simulink model "kalman_filter_state_est"  (R2024a)
settings: Solver=VariableStepAuto  StartTime=0.0  StopTime=10.0  RelTol=1e-3
undefined symbols (not defined in the file): b, Continuous, J, K, Kc, L, R, Time
libraries: simulink x3, ctrlSharedLib x1
settings Model: Creator=Harish  LastModifiedBy=Harish

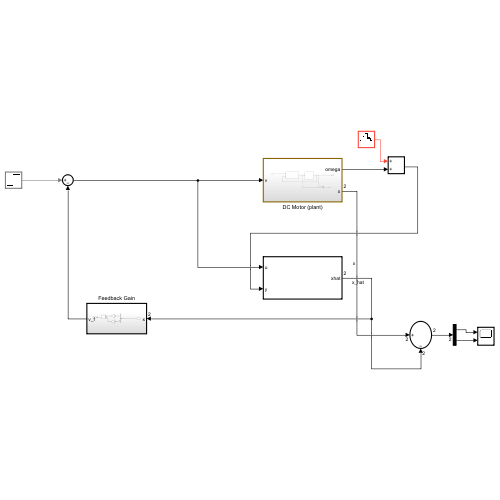
[thumbnail: Simulink's stored preview of the top-level diagram]
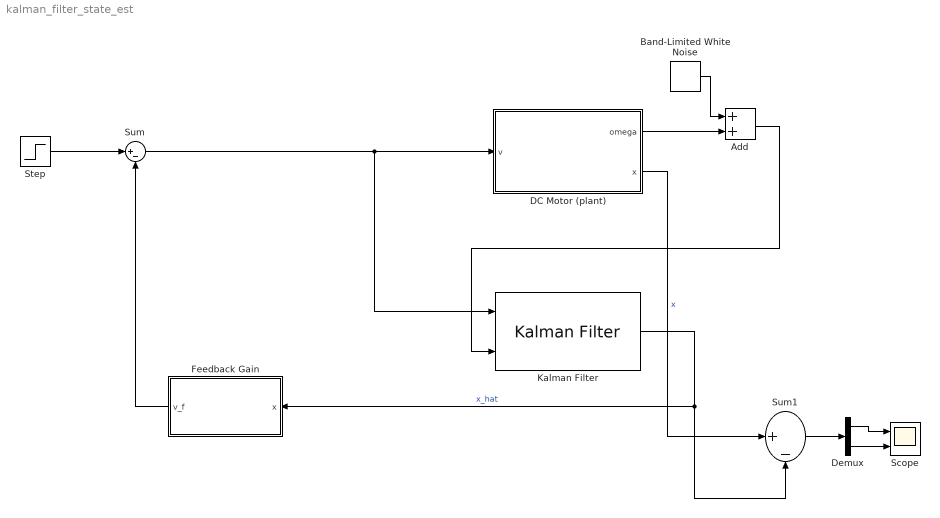
== system kalman_filter_state_est ==
  Add : Sum
  Band-Limited White Noise : simulink/Sources/Band-Limited White Noise  Cov=0.01  Ts=0.01  seed=0
  DC Motor (plant) : Subsystem
  Demux : Demux  Outputs=2
  Feedback Gain : Subsystem
  Kalman Filter : ctrlSharedLib/Kalman Filter  TimeDomain=Continuous-Time  UseCurrentEstimator=on  ModelSource=LTI State-Space Variable  ModelSourceVariable=dcMotorSS  A=0.95  B=1  C=1  D=0  NumberOfStates=1  NumberOfInputs=1  NumberOfOutputs=1  InitialEstimateSource=Dialog  X0=0  P0=10  UseK=off  UseGH=off  NumberOfProcessNoiseInputs=1  G=1  TimeInvariantG=on  H=0  TimeInvariantH=on  Q=10  TimeInvariantQ=on  R=1  TimeInvariantR=on  N=0  TimeInvariantN=on  AddInputPort=on  AddEnablePort=off  OutputEstimatedY=off  OutputP=off  Ts=-1
  Scope : Scope  NumInputPorts=2
  Step : Step  SampleTime=0
  Sum : Sum  Inputs=|+-
  Sum1 : Sum  Inputs=|+-
  wires:
  DC Motor (plant)/1(omega) -> Add/2
  Step/1 -> Sum/1
  Feedback Gain/1(v_f) -> Sum/2
  Kalman Filter/1 -> Sum1/2, Feedback Gain/1(x)  "x_hat"
  Band-Limited White Noise/1 -> Add/1
  Add/1 -> Kalman Filter/2
  DC Motor (plant)/2(x) -> Sum1/1  "x"
  Sum/1 -> Kalman Filter/1, DC Motor (plant)/1(v)
  Sum1/1 -> Demux/1
  Demux/1 -> Scope/1
  Demux/2 -> Scope/2

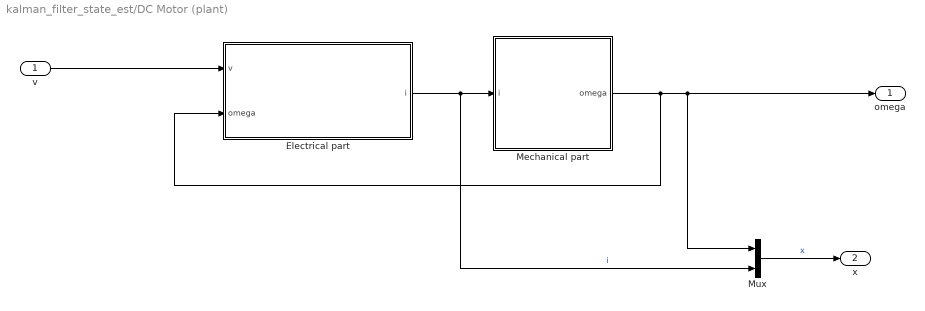
== system kalman_filter_state_est/DC Motor (plant) ==
  v : Inport
  "Electrical part " : Subsystem
  Mechanical part : Subsystem
  Mux : Mux  Inputs=2
  omega : Outport
  x : Outport  Port=2
  wires:
  "Electrical part "/1(i) -> Mux/2, Mechanical part/1(i)  "i"
  Mechanical part/1(omega) -> Mux/1, omega/1, "Electrical part "/2(omega)
  v/1 -> "Electrical part "/1(v)
  Mux/1 -> x/1  "x"

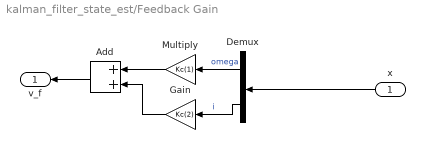
== system kalman_filter_state_est/Feedback Gain ==
  x : Inport
  Add : Sum
  Demux : Demux  Outputs=2
  Gain : Gain  Gain=Kc(2)
  Multiply : Gain  Gain=Kc(1)
  v_f : Outport
  wires:
  x/1 -> Demux/1
  Multiply/1 -> Add/1
  Add/1 -> v_f/1
  Demux/1 -> Multiply/1  "omega"
  Demux/2 -> Gain/1  "i"
  Gain/1 -> Add/2

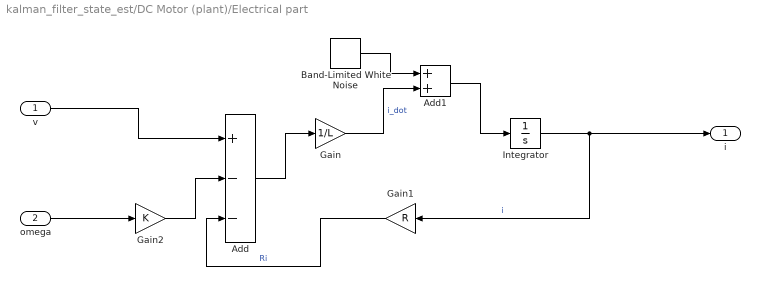
== system kalman_filter_state_est/DC Motor (plant)/Electrical part  ==
  v : Inport
  omega : Inport  Port=2
  Add : Sum  Inputs=+--
  Add1 : Sum
  Band-Limited White Noise : simulink/Sources/Band-Limited White Noise  Cov=10*0.01  Ts=0.01  seed=[23341]
  Gain : Gain  Gain=1/L
  Gain1 : Gain  Gain=R
  Gain2 : Gain  Gain=K
  Integrator : Integrator
  i : Outport
  wires:
  Add/1 -> Gain/1
  Integrator/1 -> i/1, Gain1/1  "i"
  Gain1/1 -> Add/3  "Ri"
  v/1 -> Add/1
  Gain2/1 -> Add/2
  omega/1 -> Gain2/1
  Band-Limited White Noise/1 -> Add1/1
  Gain/1 -> Add1/2  "i_dot"
  Add1/1 -> Integrator/1

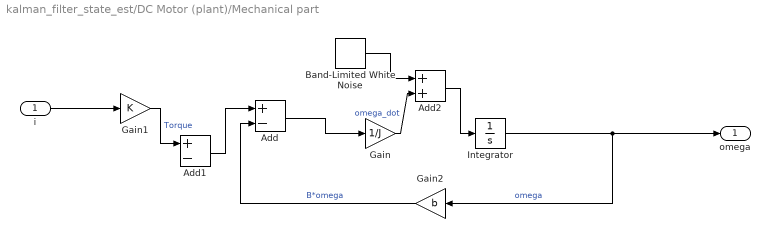
== system kalman_filter_state_est/DC Motor (plant)/Mechanical part ==
  i : Inport
  Add : Sum  Inputs=+-
  Add1 : Sum  Inputs=+-
  Add2 : Sum
  Band-Limited White Noise : simulink/Sources/Band-Limited White Noise  Cov=10*0.01  Ts=0.01  seed=25
  Gain : Gain  Gain=1/J
  Gain1 : Gain  Gain=K
  Gain2 : Gain  Gain=b
  Integrator : Integrator
  omega : Outport
  wires:
  Add/1 -> Gain/1
  Integrator/1 -> omega/1, Gain2/1  "omega"
  Gain2/1 -> Add/2  "B*omega"
  i/1 -> Gain1/1
  Gain1/1 -> Add1/1  "Torque"
  Add1/1 -> Add/1
  Band-Limited White Noise/1 -> Add2/1
  Gain/1 -> Add2/2  "omega_dot"
  Add2/1 -> Integrator/1
